simulink model "Observer_Template"  (R2020a)
settings: Solver=FixedStepAuto  StartTime=0.0  StopTime=TMax  FixedStep=DT  RelTol=1e-3
settings Model: Creator=lpwoolcock  LastModifiedBy=lpwoolcock

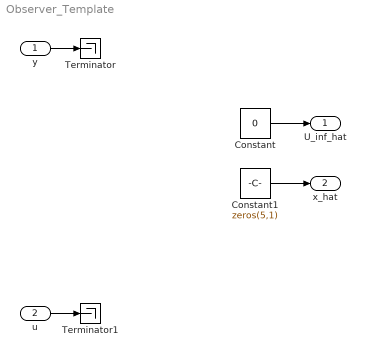
== system Observer_Template ==
  y : Inport  PortDimensions=[3 1]
  u : Inport  Port=2  PortDimensions=[2 1]
  Constant : Constant  Value=0
  Constant1 : Constant  Value=zeros(5,1)
  Terminator : Terminator
  Terminator1 : Terminator
  U_inf_hat : Outport  PortDimensions=1
  x_hat : Outport  Port=2  PortDimensions=[5 1]
  wires:
  Constant/1 -> U_inf_hat/1
  u/1 -> Terminator1/1
  y/1 -> Terminator/1
  Constant1/1 -> x_hat/1
